simulink model "ball_beam_golden_model"  (R2025b)
settings: Solver=VariableStepAuto  StartTime=0.0  StopTime=10.0  RelTol=1e-3
libraries: simulink x1
settings Model: Creator=jorda  LastModifiedBy=benja

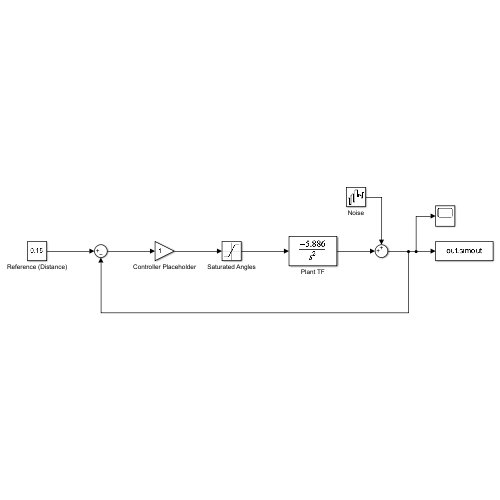
[thumbnail: Simulink's stored preview of the top-level diagram]
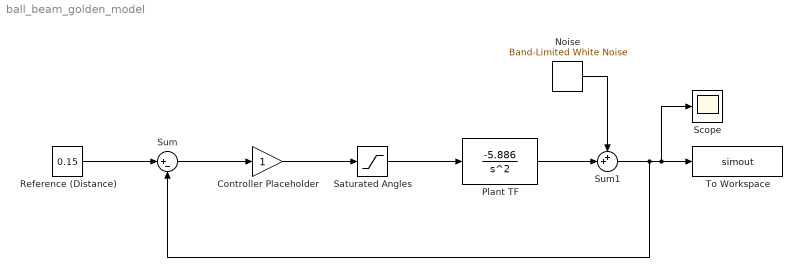
== system ball_beam_golden_model ==
  Controller Placeholder : Gain
  Noise : simulink/Sources/Band-Limited White Noise  Cov=[0.003^2]  Ts=0.026  seed=[23341]
  Plant TF : TransferFcn  Numerator=[-5.886]  Denominator=[1 0 0]
  Reference (Distance) : Constant  Value=0.15
  Saturated Angles : Saturate  UpperLimit=0.26  LowerLimit=-0.26
  Scope : Scope
      settings: ActiveDisplayYMinimum=-83.6342143273504  ActiveDisplayYMaximum=9.341711607318139
  Sum : Sum  Inputs=|+-
  Sum1 : Sum  Inputs=++|
  To Workspace : ToWorkspace  VariableName=simout  SaveFormat=Timeseries  SampleTime=-1
  wires:
  Reference (Distance)/1 -> Sum/1
  Sum/1 -> Controller Placeholder/1
  Controller Placeholder/1 -> Saturated Angles/1
  Saturated Angles/1 -> Plant TF/1
  Plant TF/1 -> Sum1/2
  Noise/1 -> Sum1/1
  Sum1/1 -> Sum/2, Scope/1, To Workspace/1
